simulink model "DC_motors"  (R2023a)
settings: Solver=VariableStepAuto  StartTime=0.0  StopTime=10.0  RelTol=1e-3
values from neighbouring files (symbols this model uses):
  d = 3e-2    (= 0.03)    [Parameters.m]
  J = (1/2)*(M * (R)^2)    (= 0.025)    [Parameters.m]
  Kb = 0.0726    [Parameters.m]
  Kt = 0.0724    [Parameters.m]
  L = 25e-2    (= 0.25)    [Parameters.m]
  La = 5.50e-6    (= 5.5e-06)    [Parameters.m]
  M = 20    [Parameters.m]
  N = 1    [Parameters.m]
  R = 5e-2    (= 0.05)    [Parameters.m]
  Ra = 4    [Parameters.m]
undefined symbols (not defined in the file or in its folder): Vl, Vr
settings Model: Creator=arnin  LastModifiedBy=arnin

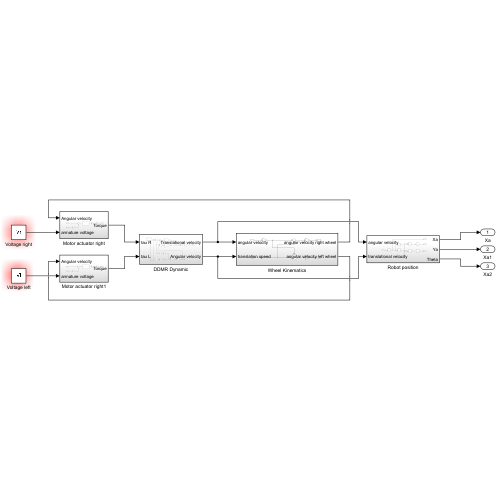
[thumbnail: Simulink's stored preview of the top-level diagram]
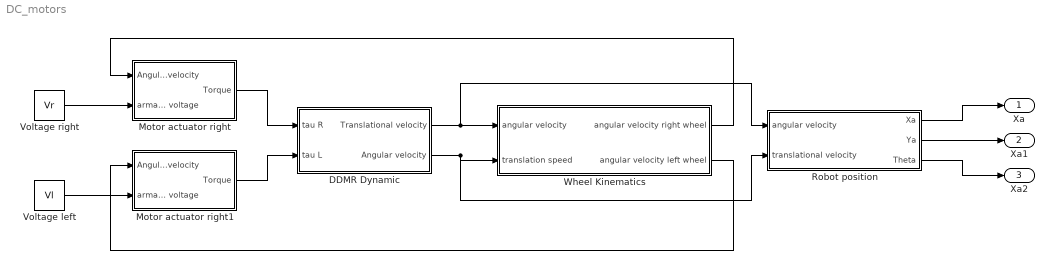
== system DC_motors ==
  DDMR Dynamic : Subsystem
  Motor actuator right : Subsystem
  Motor actuator right1 : Subsystem
  Robot position : Subsystem
  Voltage left : Constant  Value=Vl
  Voltage right : Constant  Value=Vr
  Wheel Kinematics : Subsystem
  Xa : Outport
  Xa1 : Outport  Port=2
  Xa2 : Outport  Port=3
  wires:
  Voltage right/1 -> Motor actuator right/2(armature voltage)
  Voltage left/1 -> Motor actuator right1/2(armature voltage)
  Motor actuator right/1(Torque) -> DDMR Dynamic/1(tau R)
  Motor actuator right1/1(Torque) -> DDMR Dynamic/2(tau L)
  DDMR Dynamic/1(Translational velocity) -> Robot position/1(angular velocity), Wheel Kinematics/1(angular velocity)
  DDMR Dynamic/2(Angular velocity) -> Robot position/2(translational velocity), Wheel Kinematics/2(translation speed)
  Wheel Kinematics/1(angular velocity right wheel) -> Motor actuator right/1(Angular velocity)
  Wheel Kinematics/2(angular velocity left wheel) -> Motor actuator right1/1(Angular velocity)
  Robot position/1(Xa) -> Xa/1
  Robot position/2(Ya) -> Xa1/1
  Robot position/3(Theta) -> Xa2/1

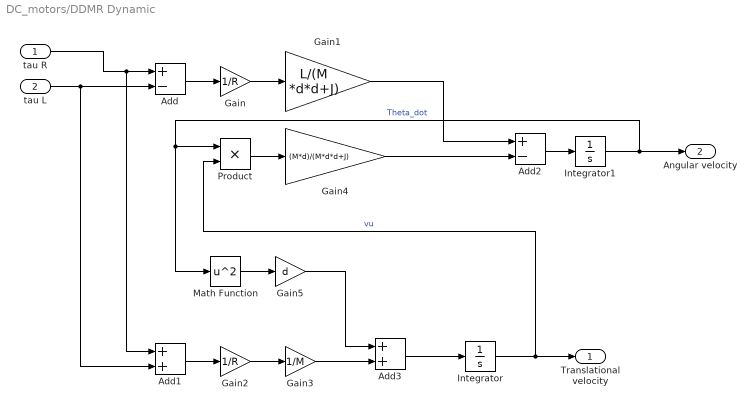
== system DC_motors/DDMR Dynamic ==
  tau R : Inport
  tau L : Inport  Port=2
  Add : Sum  Inputs=+-
  Add1 : Sum
  Add2 : Sum  Inputs=+-
  Add3 : Sum
  Gain : Gain  Gain=1/R
  Gain1 : Gain  Gain=L/(M *d*d+J)
  Gain2 : Gain  Gain=1/R
  Gain3 : Gain  Gain=1/M
  Gain4 : Gain  Gain=(M*d)/(M*d*d+J)
  Gain5 : Gain  Gain=d
  Integrator : Integrator
  Integrator1 : Integrator
  Math Function : Math  Operator=square
  Product : Product
  Translational velocity : Outport
  Angular velocity : Outport  Port=2
  wires:
  Gain4/1 -> Add2/2
  Integrator1/1 -> Math Function/1, Product/1, Angular velocity/1  "Theta_dot"
  Gain3/1 -> Add3/2
  Math Function/1 -> Gain5/1
  Gain2/1 -> Gain3/1
  Product/1 -> Gain4/1
  Integrator/1 -> Product/2, Translational velocity/1  "vu"
  Add2/1 -> Integrator1/1
  tau L/1 -> Add1/2, Add/2
  tau R/1 -> Add1/1, Add/1
  Add3/1 -> Integrator/1
  Gain5/1 -> Add3/1
  Gain1/1 -> Add2/1
  Add1/1 -> Gain2/1
  Gain/1 -> Gain1/1
  Add/1 -> Gain/1

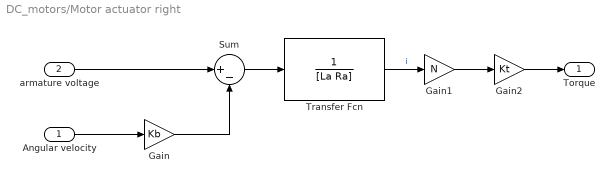
== system DC_motors/Motor actuator right ==
  Angular velocity : Inport
  armature voltage : Inport  Port=2
  Gain : Gain  Gain=Kb
  Gain1 : Gain  Gain=N
  Gain2 : Gain  Gain=Kt
  Sum : Sum  Inputs=|+-
  Transfer Fcn : TransferFcn  Denominator=[La Ra]
  Torque : Outport
  wires:
  armature voltage/1 -> Sum/1
  Angular velocity/1 -> Gain/1
  Gain/1 -> Sum/2
  Sum/1 -> Transfer Fcn/1
  Transfer Fcn/1 -> Gain1/1  "i"
  Gain1/1 -> Gain2/1
  Gain2/1 -> Torque/1

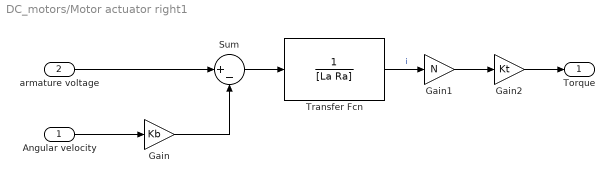
== system DC_motors/Motor actuator right1 ==
  Angular velocity : Inport
  armature voltage : Inport  Port=2
  Gain : Gain  Gain=Kb
  Gain1 : Gain  Gain=N
  Gain2 : Gain  Gain=Kt
  Sum : Sum  Inputs=|+-
  Transfer Fcn : TransferFcn  Denominator=[La Ra]
  Torque : Outport
  wires:
  armature voltage/1 -> Sum/1
  Angular velocity/1 -> Gain/1
  Gain/1 -> Sum/2
  Sum/1 -> Transfer Fcn/1
  Transfer Fcn/1 -> Gain1/1  "i"
  Gain1/1 -> Gain2/1
  Gain2/1 -> Torque/1

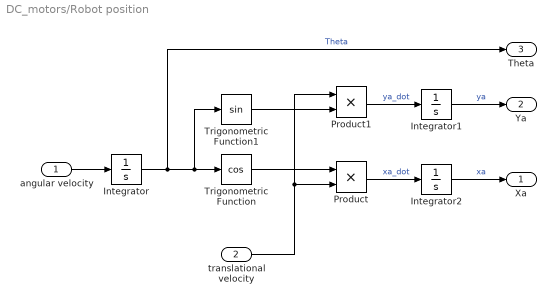
== system DC_motors/Robot position ==
  angular velocity : Inport
  translational velocity : Inport  Port=2
  Integrator : Integrator
  Integrator1 : Integrator
  Integrator2 : Integrator
  Product : Product
  Product1 : Product
  Trigonometric Function : Trigonometry  Operator=cos
  Trigonometric Function1 : Trigonometry
  Xa : Outport
  Ya : Outport  Port=2
  Theta : Outport  Port=3
  wires:
  angular velocity/1 -> Integrator/1
  Integrator/1 -> Theta/1, Trigonometric Function1/1, Trigonometric Function/1  "Theta"
  Trigonometric Function/1 -> Product/1
  Trigonometric Function1/1 -> Product1/2
  Product1/1 -> Integrator1/1  "ya_dot"
  Product/1 -> Integrator2/1  "xa_dot"
  Integrator1/1 -> Ya/1  "ya"
  Integrator2/1 -> Xa/1  "xa"
  translational velocity/1 -> Product/2, Product1/1

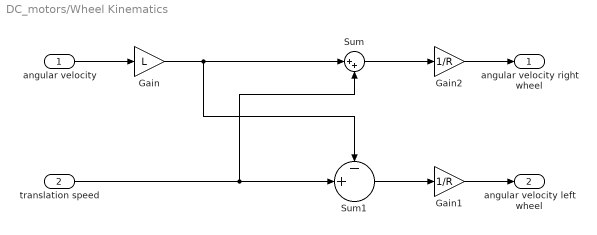
== system DC_motors/Wheel Kinematics ==
  angular velocity : Inport
  translation speed : Inport  Port=2
  Gain : Gain  Gain=L
  Gain1 : Gain  Gain=1/R
  Gain2 : Gain  Gain=1/R
  Sum : Sum  Inputs=|++
  Sum1 : Sum  Inputs=-+|
  angular velocity right wheel : Outport
  angular velocity left wheel : Outport  Port=2
  wires:
  angular velocity/1 -> Gain/1
  Gain/1 -> Sum1/1, Sum/1
  translation speed/1 -> Sum/2, Sum1/2
  Sum/1 -> Gain2/1
  Sum1/1 -> Gain1/1
  Gain1/1 -> angular velocity left wheel/1
  Gain2/1 -> angular velocity right wheel/1
